simulink model "power_accurrent"  (Simulink 6.0)
settings: Solver=VariableStepDiscrete  SolverMode=SingleTasking  StartTime=0.0  StopTime=0.5  MaxStep=1e-03  RelTol=1e-3  AbsTol=1e-6
libraries: powerlib x4
settings Model: Creator=patrice  LastModifiedBy=batserve  ExtModeTrigMode=oneshot  ExtModeArmWhenConnect=off  ExtModeAutoUpdateStatusClock=off
settings DataIOCC: LimitDataPoints=off  SignalLoggingName=sigsOut
settings OptimizationCC: BooleanDataType=off
settings DebuggingCC: SolverPrmCheckMsg=none
settings HardwareCC: TargetUnknown=on
settings RTWCC: TemplateMakefile=grt_unix.tmf

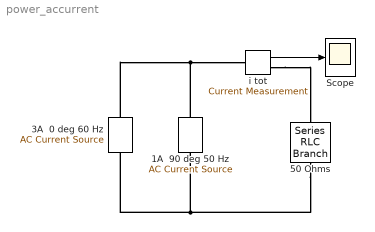
== system power_accurrent ==
  1A  90 deg 50 Hz : powerlib/Electrical Sources/AC Current Source  Orientation=up  Amplitude=1  Phase=90  Frequency=50  SampleTime=0  Measurements=None
      settings: AttributesFormatString=\n
  3A  0 deg 60 Hz : powerlib/Electrical Sources/AC Current Source  Orientation=up  Amplitude=3  Phase=0  Frequency=60  SampleTime=0  Measurements=None
      settings: AttributesFormatString=\n
  "50 Ohms " : powerlib/Elements/Series RLC Branch  Orientation=down  PhysicalDomain=powersysdomain  SubClassName=unknown  PortType=p1  LConnTagsString=__new0  RConnTagsString=__new0  Resistance=50  Inductance=0  Capacitance=inf  Measurements=None
  Scope : Scope
      settings: TickLabels=on  TimeRange=0.5  DataFormat=Array
  i tot : powerlib/Measurements/Current Measurement  Tag=PoWeRsYsTeMmEaSuReMeNt  PhasorSimulation=off  OutputType=Magnitude  PSBequivalent=0
  wires:
  i tot/1 -> Scope/1
  connections:
  i tot/RConn1 -- "50 Ohms "/LConn1
  "50 Ohms "/RConn1 -- 3A  0 deg 60 Hz/LConn1 -- 1A  90 deg 50 Hz/LConn1
  3A  0 deg 60 Hz/RConn1 -- i tot/LConn1 -- 1A  90 deg 50 Hz/RConn1
